simulink model "chua_sim"  (R2024a)
settings: Solver=VariableStepAuto  StartTime=0.0  StopTime=t_sim  RelTol=1e-3
values from neighbouring files (symbols this model uses):
  K = place(A, B, l_des)    [ChuaFL.m]    (also in chuaFLUnexact.m)
settings Model: Creator=lorenzo  LastModifiedBy=lorenzo

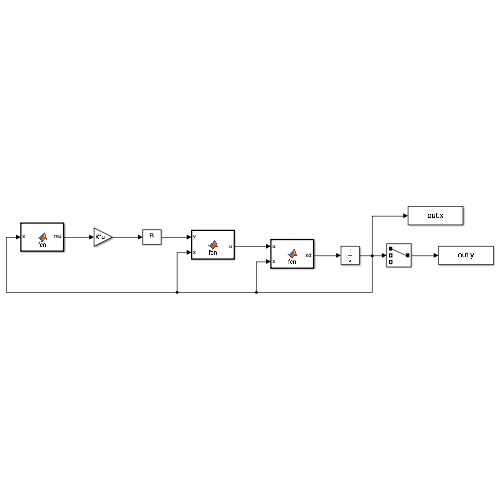
[thumbnail: Simulink's stored preview of the top-level diagram]
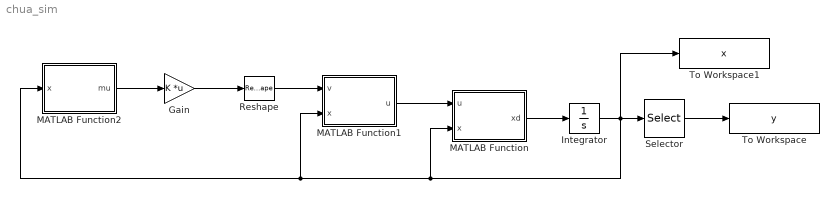
== system chua_sim ==
  Gain : Gain  Gain=K  Multiplication=Matrix(K*u)
  Integrator : Integrator
  MATLAB Function : MATLAB Function  TreatAsAtomicUnit=on
  MATLAB Function1 : MATLAB Function  TreatAsAtomicUnit=on
  MATLAB Function2 : MATLAB Function  TreatAsAtomicUnit=on
  Reshape : Reshape  OutputDimensionality=Customize  OutputDimensions=[1]
  Selector : Selector  InputPortWidth=3  IndexOptions=Index vector (dialog)  Indices=1  OutputSizes=1
  To Workspace : ToWorkspace  VariableName=y  SaveFormat=Timeseries  SampleTime=-1
  To Workspace1 : ToWorkspace  VariableName=x  SaveFormat=Timeseries  SampleTime=-1
  wires:
  MATLAB Function/1(xd) -> Integrator/1
  Integrator/1 -> To Workspace1/1, MATLAB Function1/2(x), MATLAB Function2/1(x), MATLAB Function/2(x), Selector/1
  Selector/1 -> To Workspace/1
  MATLAB Function1/1(u) -> MATLAB Function/1(u)
  MATLAB Function2/1(mu) -> Gain/1
  Gain/1 -> Reshape/1
  Reshape/1 -> MATLAB Function1/1(v)

== matlab function chua_sim/MATLAB Function ==
  data: u input; xd output; x input
function xd = fcn(u,x)

R = 0.1; alpha = 10.4; beta = 16.5;
rho = -1.16*x(1) + 0.041*x(1)^3;

xd = [alpha*(x(2)-x(1)-rho);
    x(1)-x(2)+x(3)+u;
    -beta*x(2)-R*x(3)];

== matlab function chua_sim/MATLAB Function2 ==
  data: x input; mu output
function mu = fcn(x)

alpha = 10.4;
rho = -1.16*x(1) + 0.041*x(1)^3;
mu = [x(1); alpha*(x(2)-x(1)-rho)];

== matlab function chua_sim/MATLAB Function1 ==
  data: v input; u output; x input
function u = fcn(v,x)

alpha = 10.4;
rho = -1.16*x(1) + 0.041*x(1)^3;
rhod = (123*x(1)^2)/1000 - 29/25;

u = v/alpha - (x(1)-x(2)+x(3)-alpha*(x(2)-x(1)-rho)*(1+rhod));
